simulink model "SML_HJB_Inventory"  (R2018b)
settings: Solver=VariableStepAuto  StartTime=0.0  StopTime=500  RelTol=1e-3
values from neighbouring files (symbols this model uses):
  alpha_t = 10    [HJB_Inventory.m]
  beta_t = 0.1    [HJB_Inventory.m]
  h1 = 2    [HJB_Inventory.m]
  h2 = 3    [HJB_Inventory.m]
  r = 2    [HJB_Inventory.m]
  rho = 0.01    [HJB_Inventory.m]
  theta = 0.01    [HJB_Inventory.m]
  x0 = 10    [HJB_Inventory.m]
settings Model: Creator=user  LastModifiedBy=user
settings SolverCC: ZeroCrossAlgorithm=Adaptive
settings DebuggingCC: IgnoredZcDiagnostic=none

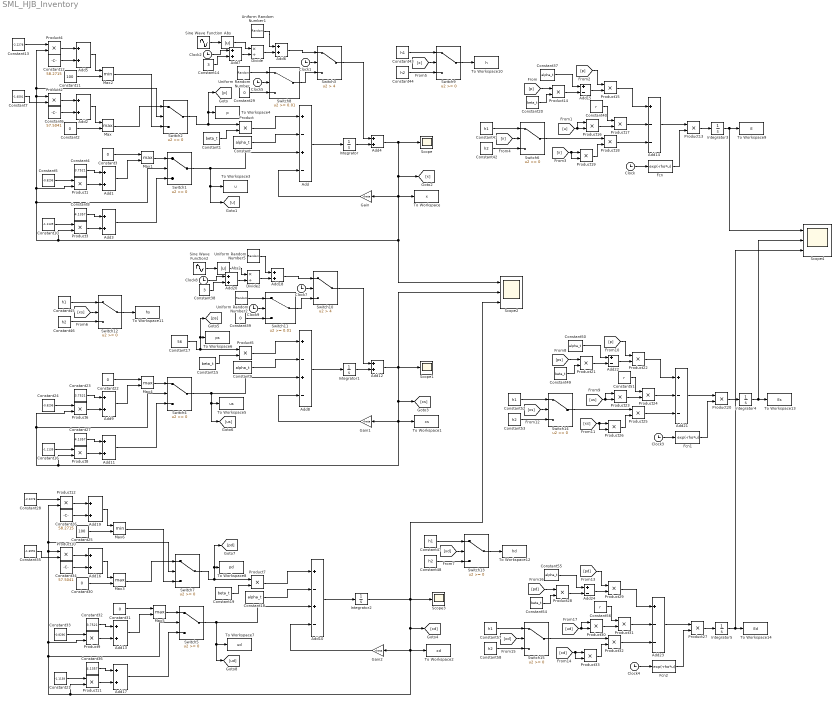
== system SML_HJB_Inventory ==
  Abs : Abs
  Abs2 : Abs
  Add : Sum  Inputs=+-+-
  Add{1..7,9,11..13,16..20} (16 alike) : Sum
  Add10 : Sum  Inputs=+-+-
  Add14 : Sum  Inputs=+--
  Add15 : Sum  Inputs=+-
  Add21 : Sum  Inputs=+--
  Add22 : Sum  Inputs=+-
  Add23 : Sum  Inputs=+--
  Add24 : Sum  Inputs=+-
  Add8 : Sum  Inputs=+-+-
  Clock{,1..5,7..9} (9 alike) : Clock
  Constant{,9,18,37,50,55} (6 alike) : Constant  Value=alpha_t
  Constant{1,15,19..20,49,54} (6 alike) : Constant  Value=beta_t
  Constant10 : Constant  Value=-1.1139
  Constant11 : Constant  Value=100
  Constant12 : Constant  Value=58.2715
  Constant13 : Constant  Value=-2.2278
  Constant14 : Constant  Value=3
  Constant16 : Constant  Value=-1.1139
  Constant17 : Constant  Value=56
  Constant{2..3,22,29..31,39} (7 alike) : Constant  Value=0
  Constant21 : Constant  Value=-1.1139
  Constant23 : Constant  Value=3.7521
  Constant24 : Constant  Value=-0.8296
  Constant25 : Constant  Value=100
  Constant26 : Constant  Value=58.2715
  Constant27 : Constant  Value=4.1357
  Constant28 : Constant  Value=-2.2278
  Constant32 : Constant  Value=3.7521
  Constant33 : Constant  Value=-0.8296
  Constant34 : Constant  Value=57.5041
  Constant35 : Constant  Value=-1.6591
  Constant36 : Constant  Value=4.1357
  Constant38 : Constant  Value=3
  Constant4 : Constant  Value=3.7521
  Constant40 : Constant  Value=r
  Constant{41,43,45,47,52,57} (6 alike) : Constant  Value=h1
  Constant{42,44,46,48,53,58} (6 alike) : Constant  Value=h2
  Constant5 : Constant  Value=-0.8296
  Constant51 : Constant  Value=r
  Constant56 : Constant  Value=r
  Constant6 : Constant  Value=57.5041
  Constant7 : Constant  Value=-1.6591
  Constant8 : Constant  Value=4.1357
  Divide : Product  Inputs=*/
  Divide2 : Product  Inputs=*/
  Fcn : Fcn  Expr=exp(-rho*u)
  Fcn1 : Fcn  Expr=exp(-rho*u)
  Fcn2 : Fcn  Expr=exp(-rho*u)
  Gain : Gain  Gain=theta
  Gain1 : Gain  Gain=theta
  Gain2 : Gain  Gain=theta
  Integrator : Integrator  InitialCondition=x0
  Integrator1 : Integrator  InitialCondition=x0
  Integrator2 : Integrator  InitialCondition=x0
  Integrator3 : Integrator
  Integrator4 : Integrator
  Integrator5 : Integrator
  Max{,1,3..5} (5 alike) : MinMax  Function=max  Inputs=2
  Max2 : MinMax  Inputs=2
  Max6 : MinMax  Inputs=2
  Product{,1..33} (34 alike) : Product
  Scope : Scope
  Scope1 : Scope
  Scope2 : Scope  NumInputPorts=3
  Scope3 : Scope
  Scope4 : Scope  NumInputPorts=3
  Sine Wave Function : Sin  SampleTime=0
  Sine Wave Function2 : Sin  SampleTime=0
  Switch{1..2,4..7,9,12..15} (11 alike) : Switch
  Switch10 : Switch  Criteria=u2 > Threshold  Threshold=4
  Switch11 : Switch  Threshold=0.01
  Switch3 : Switch  Criteria=u2 > Threshold  Threshold=4
  Switch8 : Switch  Threshold=0.01
  To Workspace : ToWorkspace  VariableName=x  SampleTime=0.01
  To Workspace1 : ToWorkspace  VariableName=xs  SampleTime=0.01
  To Workspace10 : ToWorkspace  VariableName=h  SampleTime=0.01
  To Workspace11 : ToWorkspace  VariableName=hs  SampleTime=0.01
  To Workspace12 : ToWorkspace  VariableName=hd  SampleTime=0.01
  To Workspace13 : ToWorkspace  VariableName=Es  SampleTime=0.01
  To Workspace14 : ToWorkspace  VariableName=Ed  SampleTime=0.01
  To Workspace2 : ToWorkspace  VariableName=xd  SampleTime=0.01
  To Workspace3 : ToWorkspace  VariableName=u  SampleTime=0.01
  To Workspace4 : ToWorkspace  VariableName=p  SampleTime=0.01
  To Workspace5 : ToWorkspace  VariableName=us  SampleTime=0.01
  To Workspace6 : ToWorkspace  VariableName=ps  SampleTime=0.01
  To Workspace7 : ToWorkspace  VariableName=ud  SampleTime=0.01
  To Workspace8 : ToWorkspace  VariableName=pd  SampleTime=0.01
  To Workspace9 : ToWorkspace  VariableName=E  SampleTime=0.01
  Uniform Random Number : UniformRandomNumber  Minimum=-0.2  Maximum=0.1  SampleTime=0.3
  Uniform Random Number1 : UniformRandomNumber  Minimum=-0.01  Maximum=0.01  SampleTime=0.5
  Uniform Random Number2 : UniformRandomNumber  Minimum=-0.2  Maximum=0.1  SampleTime=0.3
  Uniform Random Number5 : UniformRandomNumber  Minimum=-0.01  Maximum=0.01  SampleTime=0.5
  wires:
  Constant1/1 -> Product/2
  Sine Wave Function/1 -> Abs/1
  Add/1 -> Integrator/1
  Constant2/1 -> Max/2
  Constant3/1 -> Max1/1
  Add1/1 -> Max1/2
  Product1/1 -> Add1/2
  Constant4/1 -> Add1/1
  Constant5/1 -> Product1/1
  Product2/1 -> Add2/1
  Constant6/1 -> Add2/2
  Constant7/1 -> Product2/2
  Add2/1 -> Max/1
  Abs/1 -> Divide/1
  Max1/1 -> Switch1/1
  Constant10/1 -> Product3/1
  Constant8/1 -> Add3/1
  Product3/1 -> Add3/2
  Add3/1 -> Switch1/3
  Switch2/1 -> To Workspace4/1, [p], Product/1
  Add5/1 -> Max2/1
  Constant12/1 -> Add5/2
  Product4/1 -> Add5/1
  Constant11/1 -> Max2/2
  Constant13/1 -> Product4/1
  Max/1 -> Switch2/1
  Max2/1 -> Switch2/3
  Gain/1 -> Add/4
  Product/1 -> Add/1
  Constant/1 -> Add/2
  Switch1/1 -> [u], To Workspace3/1, Add/3
  Integrator/1 -> Add4/2
  Add4/1 -> [x], Product3/2, Switch1/2, Product2/1, Product4/2, Switch2/2, Product1/2, Scope2/1, Gain/1, To Workspace/1, Scope/1
  Switch3/1 -> Add4/1
  Clock1/1 -> Switch3/2
  Clock2/1 -> Add7/1
  Add7/1 -> Divide/2
  Constant14/1 -> Add7/2
  Divide/1 -> Add6/2
  Add6/1 -> Switch3/1
  Add12/1 -> Scope2/2, Scope1/1, [xs], To Workspace1/1, Gain1/1, Product6/2, Switch4/2, Product8/2
  Integrator1/1 -> Add12/2
  Switch4/1 -> [us], To Workspace5/1, Add8/3
  Constant9/1 -> Add8/2
  Product5/1 -> Add8/1
  Gain1/1 -> Add8/4
  Constant17/1 -> [ps], To Workspace6/1, Product5/1
  Add11/1 -> Switch4/3
  Product8/1 -> Add11/2
  Constant27/1 -> Add11/1
  Constant16/1 -> Product8/1
  Max4/1 -> Switch4/1
  Constant24/1 -> Product6/1
  Constant23/1 -> Add9/1
  Product6/1 -> Add9/2
  Add9/1 -> Max4/2
  Constant22/1 -> Max4/1
  Add8/1 -> Integrator1/1
  Constant15/1 -> Product5/2
  Integrator2/1 -> Scope2/3, Scope3/1, [xd], To Workspace2/1, Gain2/1, Product9/2, Switch7/2, Product12/2, Product10/1, Switch5/2, Product11/2
  Switch5/1 -> [ud], To Workspace7/1, Add10/3
  Constant18/1 -> Add10/2
  Product7/1 -> Add10/1
  Gain2/1 -> Add10/4
  Max6/1 -> Switch7/3
  Max3/1 -> Switch7/1
  Constant28/1 -> Product12/1
  Constant25/1 -> Max6/2
  Product12/1 -> Add19/1
  Constant26/1 -> Add19/2
  Add19/1 -> Max6/1
  Switch7/1 -> [pd], To Workspace8/1, Product7/1
  Add17/1 -> Switch5/3
  Product11/1 -> Add17/2
  Constant36/1 -> Add17/1
  Constant21/1 -> Product11/1
  Max5/1 -> Switch5/1
  Add16/1 -> Max3/1
  Constant35/1 -> Product10/2
  Constant34/1 -> Add16/2
  Product10/1 -> Add16/1
  Constant33/1 -> Product9/1
  Constant32/1 -> Add13/1
  Product9/1 -> Add13/2
  Add13/1 -> Max5/2
  Constant31/1 -> Max5/1
  Constant30/1 -> Max3/2
  Add10/1 -> Integrator2/1
  Constant19/1 -> Product7/2
  Switch8/1 -> Switch3/3
  Clock5/1 -> Switch8/2
  Constant29/1 -> Switch8/3
  Constant39/1 -> Switch11/3
  Clock9/1 -> Switch11/2
  Uniform Random Number2/1 -> Switch11/1
  Switch11/1 -> Switch10/3
  Add18/1 -> Switch10/1
  Uniform Random Number5/1 -> Add18/1
  Divide2/1 -> Add18/2
  Constant38/1 -> Add20/2
  Add20/1 -> Divide2/2
  Clock8/1 -> Add20/1
  Clock7/1 -> Switch10/2
  Abs2/1 -> Divide2/1
  Sine Wave Function2/1 -> Abs2/1
  Switch10/1 -> Add12/1
  Uniform Random Number/1 -> Switch8/1
  Uniform Random Number1/1 -> Add6/1
  Add14/1 -> Product13/1
  Fcn/1 -> Product13/2
  [p] -> Product14/1
  Product14/1 -> Add15/2
  Constant20/1 -> Product14/2
  Constant37/1 -> Add15/1
  Add15/1 -> Product15/2
  [p] -> Product15/1
  Product15/1 -> Add14/1
  Product17/1 -> Add14/2
  [u] -> Product16/1, Product16/2
  Product16/1 -> Product17/2
  Constant40/1 -> Product17/1
  Product18/1 -> Add14/3
  Switch6/1 -> Product18/1
  Product19/1 -> Product18/2
  [x] -> Product19/2, Product19/1
  [x] -> Switch6/2
  Constant41/1 -> Switch6/1
  Constant42/1 -> Switch6/3
  Product13/1 -> Integrator3/1
  Integrator3/1 -> Scope4/1, To Workspace9/1
  Constant44/1 -> Switch9/3
  Constant43/1 -> Switch9/1
  [x] -> Switch9/2
  Switch9/1 -> To Workspace10/1
  Constant46/1 -> Switch12/3
  Switch12/1 -> To Workspace11/1
  Constant45/1 -> Switch12/1
  [xs] -> Switch12/2
  [xd] -> Switch13/2
  Constant47/1 -> Switch13/1
  Switch13/1 -> To Workspace12/1
  Constant48/1 -> Switch13/3
  Clock/1 -> Fcn/1
  Clock3/1 -> Fcn1/1
  Integrator4/1 -> Scope4/2, To Workspace13/1
  Product20/1 -> Integrator4/1
  Constant53/1 -> Switch14/3
  Constant52/1 -> Switch14/1
  [xs] -> Switch14/2
  [xs] -> Product26/1, Product26/2
  Product26/1 -> Product25/2
  Switch14/1 -> Product25/1
  Product25/1 -> Add21/3
  Constant51/1 -> Product24/1
  Product23/1 -> Product24/2
  [us] -> Product23/2, Product23/1
  Product24/1 -> Add21/2
  Product22/1 -> Add21/1
  [p] -> Product22/1
  Add22/1 -> Product22/2
  Constant50/1 -> Add22/1
  Constant49/1 -> Product21/2
  Product21/1 -> Add22/2
  [ps] -> Product21/1
  Fcn1/1 -> Product20/2
  Add21/1 -> Product20/1
  Add23/1 -> Product27/1
  Fcn2/1 -> Product27/2
  [pd] -> Product28/1
  Product28/1 -> Add24/2
  Constant54/1 -> Product28/2
  Constant55/1 -> Add24/1
  Add24/1 -> Product29/2
  [pd] -> Product29/1
  Product29/1 -> Add23/1
  Product31/1 -> Add23/2
  [ud] -> Product30/1, Product30/2
  Product30/1 -> Product31/2
  Constant56/1 -> Product31/1
  Product32/1 -> Add23/3
  Switch15/1 -> Product32/1
  Product33/1 -> Product32/2
  [xd] -> Product33/2, Product33/1
  [xd] -> Switch15/2
  Constant57/1 -> Switch15/1
  Constant58/1 -> Switch15/3
  Product27/1 -> Integrator5/1
  Integrator5/1 -> Scope4/3, To Workspace14/1
  Clock4/1 -> Fcn2/1
